simulink model "MIRSU"  (R2023b)
settings: Solver=FixedStepAuto  StartTime=0.0  StopTime=7  FixedStep=0.001  RelTol=1e-3
undefined symbols (not defined in the file): A, A_d_array, B, B_d_array, C, D, disc_intervals
settings Model: Creator=drafty  LastModifiedBy=drafty

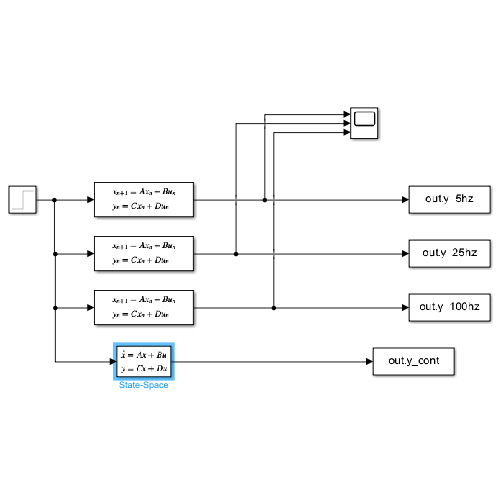
[thumbnail: Simulink's stored preview of the top-level diagram]
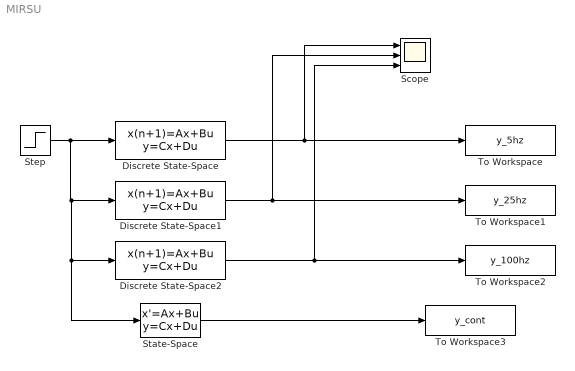
== system MIRSU ==
  Discrete State-Space : DiscreteStateSpace  A=A_d_array{1}  B=B_d_array{1}  C=[0 1 1]  D=[0]  SampleTime=disc_intervals(1)
  Discrete State-Space1 : DiscreteStateSpace  A=A_d_array{2}  B=B_d_array{2}  C=[0 1 1]  D=[0]  SampleTime=disc_intervals(2)
  Discrete State-Space2 : DiscreteStateSpace  A=A_d_array{3}  B=B_d_array{3}  C=[0 1 1]  D=[0]  SampleTime=disc_intervals(3)
  Scope : Scope  NumInputPorts=3
  State-Space : StateSpace  A=A  B=B  C=C  D=D  InitialCondition=0
  Step : Step  Time=0  SampleTime=0
  To Workspace : ToWorkspace  VariableName=y_5hz  SaveFormat=Timeseries  SampleTime=-1
  To Workspace1 : ToWorkspace  VariableName=y_25hz  SaveFormat=Timeseries  SampleTime=-1
  To Workspace2 : ToWorkspace  VariableName=y_100hz  SaveFormat=Timeseries  SampleTime=-1
  To Workspace3 : ToWorkspace  VariableName=y_cont  SaveFormat=Timeseries  SampleTime=-1
  wires:
  Step/1 -> State-Space/1, Discrete State-Space2/1, Discrete State-Space1/1, Discrete State-Space/1
  Discrete State-Space/1 -> Scope/1, To Workspace/1
  Discrete State-Space2/1 -> Scope/3, To Workspace2/1
  Discrete State-Space1/1 -> To Workspace1/1, Scope/2
  State-Space/1 -> To Workspace3/1
